simulink model "DynamicModelingAres"  (R2018a)
settings: Solver=VariableStepAuto  StartTime=0.0  StopTime=155.0  RelTol=1e-3
libraries: dspmtrx3 x5, shared6dof x1, aerolibatmos2 x1
settings Model: Creator=Alex  LastModifiedBy=Alex

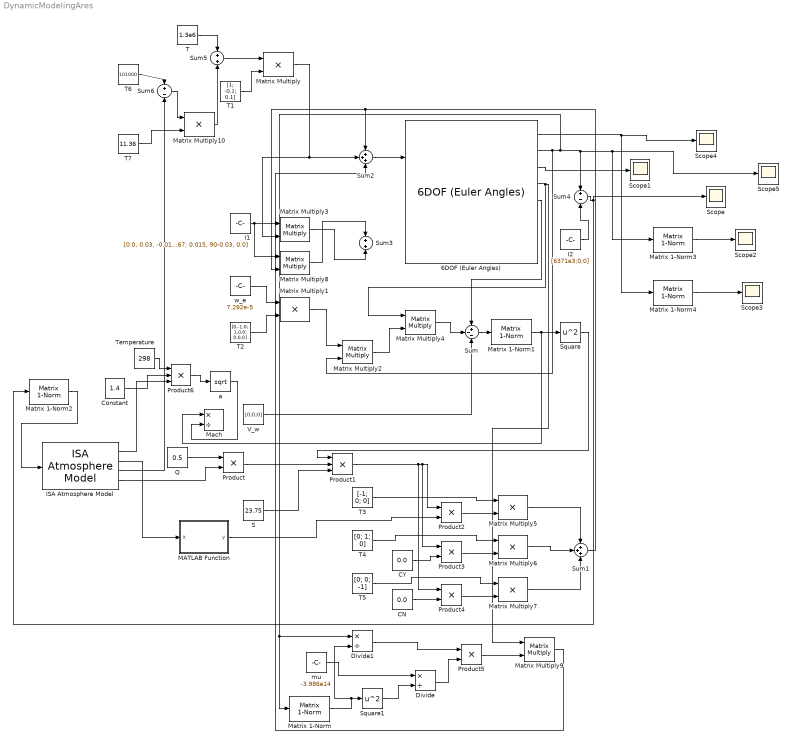
== system DynamicModelingAres ==
  6DOF (Euler Angles) : shared6dof/6DOF (Euler Angles)  units=Metric (MKS)  mtype=Fixed  rep=Quaternion  xme_0=[6371e3 0 0]  Vm_0=[0 464 0]  eul_0=[0 0 0]  pm_0=[0 0 0]  mass_0=2.54e4  mass_e=0.5  mass_f=2.0  inertia=[1.71e6, -2.15e3, 7.48e4; -2.15e3, 3.9e8, -2.06e3; 7.48e4, -2.06e3, 3.9e8]  inertia_e=eye(3)  inertia_f=2*eye(3)  k_quat=1.0  vre_flag=on  abi_flag=off  aMode=0
      settings: SourceProductBaseCode=AE
  CN : Constant  Value=0.0  VectorParams1D=off
  CY : Constant  Value=0.0  VectorParams1D=off
  Constant : Constant  Value=1.4
  Divide : Product  Inputs=*/
  Divide1 : Product  Inputs=*/
  I1 : Constant  Value=[0.0, 0.03, -0.015; -0.03, 0.0, -90+67; 0.015, 90-0.03, 0.0]  VectorParams1D=off
  I2 : Constant  Value=[6371e3;0;0]  VectorParams1D=off
  ISA Atmosphere Model : aerolibatmos2/ISA Atmosphere Model  custom=off  g=9.80665  gamma=1.4  R=287.0531  L=0.0065  h_trop=11000  h_strat=20000  rho0=1.225  P0=101325  T0=288.15  h0=0
      settings: SourceProductName=Aerospace Blockset
  MATLAB Function : MATLAB Function  TreatAsAtomicUnit=on
  Mach : Product  Inputs=*/
  Matrix 1-Norm{,1..4} (5 alike) : dspmtrx3/Matrix  1-Norm  roundingMode=Floor  overflowMode=off  outputDataTypeStr=Inherit: Same as accumulator  outputMin=[]  outputMax=[]  outputLastDataTypeStr=Inherit: Same as accumulator
      settings: SourceProductName=DSP System Toolbox  SourceProductBaseCode=DS
  Matrix Multiply{,1,5..7,10} (6 alike) : Product
  Matrix Multiply{2..4,8..9} (5 alike) : Product  Multiplication=Matrix(*)
  Product{,2..5} (5 alike) : Product
  Product1 : Product  Inputs=3
  Product6 : Product  Inputs=3
  Q : Constant  Value=0.5  VectorParams1D=off
  S : Constant  Value=23.75  VectorParams1D=off
  Scope{,1..5} (6 alike) : Scope
  Square : Math  Operator=square  SaturateOnIntegerOverflow=on
  Square1 : Math  Operator=square  SaturateOnIntegerOverflow=on
  Sum : Sum  Inputs=+--
  Sum1 : Sum  Inputs=+++
  Sum2 : Sum  Inputs=+++
  Sum3 : Sum
  Sum4 : Sum  Inputs=+-
  Sum5 : Sum
  Sum6 : Sum  Inputs=+-
  T : Constant  Value=1.3e6
  T1 : Constant  Value=[1; -0.1; 0.1]  VectorParams1D=off
  T2 : Constant  Value=[0,-1,0; 1,0,0; 0,0,0]  VectorParams1D=off
  T3 : Constant  Value=[-1; 0; 0]  VectorParams1D=off
  T4 : Constant  Value=[0; 1; 0]  VectorParams1D=off
  T5 : Constant  Value=[0; 0; -1]  VectorParams1D=off
  T6 : Constant  Value=101000
  T7 : Constant  Value=11.36
  "Temperature " : Constant  Value=298
  V_w : Constant  Value=[0;0;0]  VectorParams1D=off
  a : Sqrt  SaturateOnIntegerOverflow=on
  mu : Constant  Value=-3.986e14  VectorParams1D=off
  w_e : Constant  Value=7.292e-5  VectorParams1D=off
  wires:
  Matrix Multiply/1 -> Sum2/2, Matrix Multiply3/2
  T1/1 -> Matrix Multiply/2
  I1/1 -> Matrix Multiply8/1, Matrix Multiply3/1
  w_e/1 -> Matrix Multiply1/1
  T2/1 -> Matrix Multiply1/2
  Matrix Multiply1/1 -> Matrix Multiply2/1
  6DOF (Euler Angles)/4 -> Matrix Multiply9/1, Matrix Multiply4/1
  Matrix Multiply2/1 -> Matrix Multiply4/2
  6DOF (Euler Angles)/5 -> Sum/1
  Matrix Multiply4/1 -> Sum/2
  V_w/1 -> Sum/3
  S/1 -> Product1/3
  Square/1 -> Product1/1
  CN/1 -> Product4/2
  CY/1 -> Product3/2
  Product1/1 -> Product4/1, Product3/1, Product2/1
  T3/1 -> Matrix Multiply5/1
  Product2/1 -> Matrix Multiply5/2
  T4/1 -> Matrix Multiply6/1
  Product3/1 -> Matrix Multiply6/2
  T5/1 -> Matrix Multiply7/1
  Product4/1 -> Matrix Multiply7/2
  Sum1/1 -> Sum2/1, Matrix Multiply8/2
  Sum2/1 -> 6DOF (Euler Angles)/1
  Matrix Multiply3/1 -> Sum3/2
  Matrix Multiply7/1 -> Sum1/3
  Matrix Multiply6/1 -> Sum1/2
  Matrix Multiply5/1 -> Sum1/1
  6DOF (Euler Angles)/2 -> Matrix Multiply2/2, Scope5/1, Matrix 1-Norm3/1, Sum4/1, Matrix 1-Norm/1, Divide1/1
  mu/1 -> Divide/1
  Square1/1 -> Divide/2
  Divide/1 -> Product5/2
  Divide1/1 -> Product5/1
  Sum4/1 -> Matrix 1-Norm2/1, Scope/1
  I2/1 -> Sum4/2
  Product5/1 -> Matrix Multiply9/2
  Matrix 1-Norm/1 -> Square1/1, Divide1/2
  Sum/1 -> Matrix 1-Norm1/1
  Matrix 1-Norm1/1 -> Mach/1, Square/1
  Matrix Multiply8/1 -> Sum3/1
  Matrix Multiply9/1 -> Sum2/3
  6DOF (Euler Angles)/3 -> Scope1/1
  MATLAB Function/1(y) -> Product2/2
  Q/1 -> Product/1
  Product/1 -> Product1/2
  "Temperature "/1 -> Product6/1
  Product6/1 -> a/1
  Constant/1 -> Product6/2
  a/1 -> Mach/2
  Matrix 1-Norm2/1 -> ISA Atmosphere Model/1
  ISA Atmosphere Model/1 -> Product6/3
  ISA Atmosphere Model/4 -> Product/2
  ISA Atmosphere Model/2 -> MATLAB Function/1(x)
  T/1 -> Sum5/1
  Sum5/1 -> Matrix Multiply/1
  T6/1 -> Sum6/1
  ISA Atmosphere Model/3 -> Sum6/2
  T7/1 -> Matrix Multiply10/2
  Sum6/1 -> Matrix Multiply10/1
  Matrix Multiply10/1 -> Sum5/2
  Matrix 1-Norm3/1 -> Scope2/1
  6DOF (Euler Angles)/1 -> Scope4/1, Matrix 1-Norm4/1
  Matrix 1-Norm4/1 -> Scope3/1

== matlab function DynamicModelingAres/MATLAB Function ==
  data: x input; y output
function y = fcn(x)

if x < 0.6
    y = 0.51;
elseif x > 2.5
    y = 0.37;
else
    y = -0.879933*x*x + 2.60687*x - 0.6529;
end
